simulink model "Quadrotor_two_blocks"  (R2020a)
settings: Solver=FixedStepAuto  StartTime=0.0  StopTime=options.T_train  FixedStep=options.dt  RelTol=1e-6
undefined symbols (not defined in the file or in its folder): options, Quad
libraries: neural x205, simulink x3
(part 7 of 14)

== system Quadrotor_two_blocks/NN/Layer 3/Delays 1 ==
  "p{3}" : Inport  PortDimensions=30
      mask Display: e = 0.06;c1 = [120 230 180]/255;c2 = ([120 230 180]+0)/(256+128);c3 = ([120 230 180]+128)/(256+128);patch([0 1 1 0],[0 0 1 1],c1);patch([0 1 1 1-e 1-e 0+e],[0 0 1 1-e 0+e 0+e],c2);patch([0 0 1 1-e 0+e 0+e],[0 1 1 1-e 1-e 0+e],c3);plot([0 1 1 0 0],[0 0 1 1 0]);
  mux : Mux  Inputs=1
      mask Display: e = 0.06;c1 = [120 150 230]/255;c2 = ([120 150 230]+0)/383;c3 = ([120 150 230]+128)/383;patch([0 1 1 0],[0 0 1 1],c1);patch([0 1 1 1-e 1-e 0+e],[0 0 1 1-e 0+e 0+e],c2);patch([0 0 1 1-e 0+e 0+e],[0 1 1 1-e 1-e 0+e],c3);plot([0 1 1 0 0],[0 0 1 1 0]);disp('Mux')
  "pd{3,2}" : Outport
      mask Display: e = 0.06;c1 = [120 230 180]/255;c2 = ([120 230 180]+0)/(256+128);c3 = ([120 230 180]+128)/(256+128);patch([0 1 1 0],[0 0 1 1],c1);patch([0 1 1 1-e 1-e 0+e],[0 0 1 1-e 0+e 0+e],c2);patch([0 0 1 1-e 0+e 0+e],[0 1 1 1-e 1-e 0+e],c3);plot([0 1 1 0 0],[0 0 1 1 0]);
  wires:
  "p{3}"/1 -> mux/1
  mux/1 -> "pd{3,2}"/1

== system Quadrotor_two_blocks/NN/Layer 3/LW{3,2} ==
  "ad{3,2}" : Inport  PortDimensions=30
      mask Display: e = 0.06;c1 = [120 230 180]/255;c2 = ([120 230 180]+0)/(256+128);c3 = ([120 230 180]+128)/(256+128);patch([0 1 1 0],[0 0 1 1],c1);patch([0 1 1 1-e 1-e 0+e],[0 0 1 1-e 0+e 0+e],c2);patch([0 0 1 1-e 0+e 0+e],[0 1 1 1-e 1-e 0+e],c3);plot([0 1 1 0 0],[0 0 1 1 0]);
  "IW{3,2}(1,:)'" : Constant  Value=[-0.26594083127618273199033183118444867432117462158203125;-1.0210525131770411544351873089908622205257415771484375;0.30545839861076828913866165748913772404193878173828125;0.0309919114401060909191887304814372328110039234161376953125;-0.73740963197516096183647960060625337064266204833984375;0.0615264643735852490014082150082685984671115875244140625;1.2371763220660463300504261496826075017452239990234375;-0.1340755837814512074768202865016064606606960296630859375;0.52192850814451519081416108747362159192562103271484375;0.3179660779336177522935713568585924804210662841796875;1.8557792800562189494684162127668969333171844482421875;0.440626162595649073505654769178363494575023651123046875;-0.89141442392688985396631551338941790163516998291015625;-1.40392726383320276539734550169669091701507568359375;-0.0093768808390524878426663946129338000901043415069580078125;-1.497598488042174214029955692240037024021148681640625;-0.56384143616242743402011683429009281098842620849609375;1.7827288996481580607422756656887941062450408935546875;-1.10640090799874091231913553201593458652496337890625;0.1196631980717009213766033326464821584522724151611328125;-0.1317737072209012871848443637645686976611614227294921875;0.91756967896656449479309003436355851590633392333984375;0.328089760720642775737587726325727999210357666015625;0.426380306867213842991759520373307168483734130859375;0.035794207671944633375460398383438587188720703125;0.1608528623550131708697108479100279510021209716796875;0.1790443040843421318442096890066750347614288330078125;-0.58903866560669204677225252453354187309741973876953125;0.6517385209835542259071416992810554802417755126953125;0.302190232396869207232015241970657370984554290771484375]
      mask Display: e = 0.06;c1 = [120 150 230]/255;c2 = ([120 150 230]+0)/383;c3 = ([120 150 230]+128)/383;patch([0 1 1 0],[0 0 1 1],c1);patch([0 1 1 1-e 1-e 0+e],[0 0 1 1-e 0+e 0+e],c2);patch([0 0 1 1-e 0+e 0+e],[0 1 1 1-e 1-e 0+e],c3);plot([0 1 1 0 0],[0 0 1 1 0]);disp('weights');
  "IW{3,2}(2,:)'" : Constant  Value=[0.33744474733492924034550242140539921820163726806640625;-0.2085190544035906701214599934246507473289966583251953125;-0.1255370354318803005622129376206430606544017791748046875;-0.361418338169405106707898767126607708632946014404296875;0.313141565270156296829640041323727928102016448974609375;-1.34995056245598643585026366054080426692962646484375;0.90600383742534074116292686085216701030731201171875;1.1626004424155891303627186061930842697620391845703125;0.92469037503852591353137313490151427686214447021484375;-0.87378422621586537832882868315209634602069854736328125;0.3994801343331599863262226790538989007472991943359375;0.568520195512125514625267896917648613452911376953125;-0.2688954998979180555096490934374742209911346435546875;-0.1495699709580518288465356135930051095783710479736328125;-0.232210590491328583429009313476854003965854644775390625;0.47887708266422868153000536040053702890872955322265625;0.63989105986046990182103400002233684062957763671875;-0.71735229499152219911906058769091032445430755615234375;0.55957358573511850607928863610140979290008544921875;-0.0960833035156002102095129657755023799836635589599609375;0.312934254119361987545033798596705310046672821044921875;0.156066035844688977274330454747541807591915130615234375;0.812319303498020506282273345277644693851470947265625;0.11571196090934143807515965818311087787151336669921875;0.17816550594502122972784263765788637101650238037109375;-0.383977057698982660038922176681808196008205413818359375;2.17971938370754170222198808914981782436370849609375;-0.9431413606304046570727450671256519854068756103515625;-1.0538118842752428605535897077061235904693603515625;-0.5897085269588391298611895763315260410308837890625]
      mask Display: e = 0.06;c1 = [120 150 230]/255;c2 = ([120 150 230]+0)/383;c3 = ([120 150 230]+128)/383;patch([0 1 1 0],[0 0 1 1],c1);patch([0 1 1 1-e 1-e 0+e],[0 0 1 1-e 0+e 0+e],c2);patch([0 0 1 1-e 0+e 0+e],[0 1 1 1-e 1-e 0+e],c3);plot([0 1 1 0 0],[0 0 1 1 0]);disp('weights');
  "IW{3,2}(3,:)'" : Constant  Value=[-0.6335697989043242994711135906982235610485076904296875;-0.1343776203969931637427492887582047842442989349365234375;0.2107485675079063813797120019444264471530914306640625;-0.471293797973846018134480573280598036944866180419921875;0.881101645491094043194379992200993001461029052734375;-0.395904028642520111613833933006389997899532318115234375;0.9541607331500367994436828666948713362216949462890625;1.5238431923374815557536976484698243439197540283203125;0.168828201538509692358758229602244682610034942626953125;-1.0782325865478841198097370579489506781101226806640625;-0.9878852333117651429716943312087096273899078369140625;-0.274508994125400473951259527893853373825550079345703125;-0.1388637628177754324010351183460443280637264251708984375;0.90694849334485516667569982018903829157352447509765625;-1.43628401967157603991154246614314615726470947265625;0.06002989728634845756349847079036408104002475738525390625;-0.48093683863805469780317025652038864791393280029296875;0.425134331812044574672171393103781156241893768310546875;0.469441503546212335340470644950983114540576934814453125;-1.478429577639362779706289074965752661228179931640625;1.1419798804367820022065416196710430085659027099609375;-0.2733285941165155552567966878996230661869049072265625;-0.352435777923840010128486710527795366942882537841796875;-0.285385952349365201730080343622830696403980255126953125;1.0184468524173855286107936990447342395782470703125;0.85005112270336968816053513364749960601329803466796875;-1.705206712053906503712141784490086138248443603515625;-0.15205458222841838900052380267879925668239593505859375;-0.52750830136400050918155102408491075038909912109375;-0.512993057510401140319800106226466596126556396484375]
      mask Display: e = 0.06;c1 = [120 150 230]/255;c2 = ([120 150 230]+0)/383;c3 = ([120 150 230]+128)/383;patch([0 1 1 0],[0 0 1 1],c1);patch([0 1 1 1-e 1-e 0+e],[0 0 1 1-e 0+e 0+e],c2);patch([0 0 1 1-e 0+e 0+e],[0 1 1 1-e 1-e 0+e],c3);plot([0 1 1 0 0],[0 0 1 1 0]);disp('weights');
  "IW{3,2}(4,:)'" : Constant  Value=[-0.7030552584173428432023911227588541805744171142578125;0.059140034721871841127960323092338512651622295379638671875;-0.535966910381663552698228158988058567047119140625;-0.86295558672674455014117711471044458448886871337890625;0.467161951422462473626495693679316900670528411865234375;-0.261172734141019768916436305516981519758701324462890625;-0.384149580148782920918648642327752895653247833251953125;-0.676880388613721351021013106219470500946044921875;-0.7585738181397745361067563862889073789119720458984375;-0.6207965299636233336144641725695692002773284912109375;0.490384049562948842737597487939638085663318634033203125;-0.4223820867201819595493361703120172023773193359375;0.59978784862219214346623630262911319732666015625;-0.460926197327715725382546452237875200808048248291015625;0.51874298208028479795217435821541585028171539306640625;0.93663303965249899984968351418501697480678558349609375;0.434009159105308572890180585091002285480499267578125;-0.147956401728020658925544239536975510418415069580078125;0.1067236544770215067590157786980853416025638580322265625;-0.200749063601315558269533312341081909835338592529296875;-0.11986393487109921196509532137497444637119770050048828125;-0.501579391147794151351035907282494008541107177734375;0.468814003108335930480876641013310290873050689697265625;-0.95740835901870824375947677253861911594867706298828125;-0.73345690770309401873561228057951666414737701416015625;-0.459012732540319490226465859450399875640869140625;-0.325732654870988846962376328519894741475582122802734375;0.1400587764549774683064953251232509501278400421142578125;0.1468991295227192461769760711831622757017612457275390625;-0.7553559899694894941291067880229093134403228759765625]
      mask Display: e = 0.06;c1 = [120 150 230]/255;c2 = ([120 150 230]+0)/383;c3 = ([120 150 230]+128)/383;patch([0 1 1 0],[0 0 1 1],c1);patch([0 1 1 1-e 1-e 0+e],[0 0 1 1-e 0+e 0+e],c2);patch([0 0 1 1-e 0+e 0+e],[0 1 1 1-e 1-e 0+e],c3);plot([0 1 1 0 0],[0 0 1 1 0]);disp('weights');
  Mux : Mux
      mask Display: e = 0.06;c1 = [120 150 230]/255;c2 = ([120 150 230]+0)/383;c3 = ([120 150 230]+128)/383;patch([0 1 1 0],[0 0 1 1],c1);patch([0 1 1 1-e 1-e 0+e],[0 0 1 1-e 0+e 0+e],c2);patch([0 0 1 1-e 0+e 0+e],[0 1 1 1-e 1-e 0+e],c3);plot([0 1 1 0 0],[0 0 1 1 0]);disp('Mux');
  dotprod{1..4} (4 alike) : neural/Weight Functions/dotprod
  "lz{3,2}" : Outport
      mask Display: e = 0.06;c1 = [120 230 180]/255;c2 = ([120 230 180]+0)/(256+128);c3 = ([120 230 180]+128)/(256+128);patch([0 1 1 0],[0 0 1 1],c1);patch([0 1 1 1-e 1-e 0+e],[0 0 1 1-e 0+e 0+e],c2);patch([0 0 1 1-e 0+e 0+e],[0 1 1 1-e 1-e 0+e],c3);plot([0 1 1 0 0],[0 0 1 1 0]);
  wires:
  "IW{3,2}(1,:)'"/1 -> dotprod1/1
  "ad{3,2}"/1 -> dotprod1/2, dotprod2/2, dotprod3/2, dotprod4/2
  dotprod1/1 -> Mux/1
  "IW{3,2}(2,:)'"/1 -> dotprod2/1
  dotprod2/1 -> Mux/2
  "IW{3,2}(3,:)'"/1 -> dotprod3/1
  dotprod3/1 -> Mux/3
  "IW{3,2}(4,:)'"/1 -> dotprod4/1
  dotprod4/1 -> Mux/4
  Mux/1 -> "lz{3,2}"/1

== system Quadrotor_two_blocks/NN_cex_1/Layer 1/Delays 1 ==
  "p{1}" : Inport  PortDimensions=27
      mask Display: e = 0.06;c1 = [120 230 180]/255;c2 = ([120 230 180]+0)/(256+128);c3 = ([120 230 180]+128)/(256+128);patch([0 1 1 0],[0 0 1 1],c1);patch([0 1 1 1-e 1-e 0+e],[0 0 1 1-e 0+e 0+e],c2);patch([0 0 1 1-e 0+e 0+e],[0 1 1 1-e 1-e 0+e],c3);plot([0 1 1 0 0],[0 0 1 1 0]);
  mux : Mux  Inputs=1
      mask Display: e = 0.06;c1 = [120 150 230]/255;c2 = ([120 150 230]+0)/383;c3 = ([120 150 230]+128)/383;patch([0 1 1 0],[0 0 1 1],c1);patch([0 1 1 1-e 1-e 0+e],[0 0 1 1-e 0+e 0+e],c2);patch([0 0 1 1-e 0+e 0+e],[0 1 1 1-e 1-e 0+e],c3);plot([0 1 1 0 0],[0 0 1 1 0]);disp('Mux')
  "pd{1,1}" : Outport
      mask Display: e = 0.06;c1 = [120 230 180]/255;c2 = ([120 230 180]+0)/(256+128);c3 = ([120 230 180]+128)/(256+128);patch([0 1 1 0],[0 0 1 1],c1);patch([0 1 1 1-e 1-e 0+e],[0 0 1 1-e 0+e 0+e],c2);patch([0 0 1 1-e 0+e 0+e],[0 1 1 1-e 1-e 0+e],c3);plot([0 1 1 0 0],[0 0 1 1 0]);
  wires:
  "p{1}"/1 -> mux/1
  mux/1 -> "pd{1,1}"/1
